simulink model "TargetPosVel"  (R2025a)
settings: Solver=ode4  StartTime=0.0  StopTime=stopTime  FixedStep=timeStep  RelTol=1e-3
values from neighbouring files (symbols this model uses):
  rand_vec = [0, rand(), rand()]    [model_parameters.m]
undefined symbols (not defined in the file or in its folder): angular_rate_noise_ON, angular_rate_noise_power, c, CD, dayValue, dimx, dimz, hourValue, I, I_W, IAU, K_optics, kd, kq, max_h, max_t, minuteValue, mu_E, Omega_E, Phi, pointing_body, q, quat0, quaternion_bias, quaternion_noise_ON, quaternion_sigma, R_E, rcp, res_dipole, secondValue, sma, timeStep, w0, WMM2020, yearValue
libraries: aerolibutil x19, matrix_library x10, aerolibtransform2 x8, vrlib x5, simulink x1, sharedTrackingLibrary x1, aerolibatmos2 x1, aerolibgravity2 x1, sharedtransform x1, sensorgpslib x1, visionsources x1
(part 2 of 2)

== system TargetPosVel/Main/Attiude Controller/Nadir Pointing Controller/Nadir Pointing/Subsystem ==
  r_ECI : Inport
  v_ECI : Inport  Port=2
  Cross Product : matrix_library/Cross Product
  Cross Product1 : matrix_library/Cross Product
  Gain : Gain  Gain=-1
  Matrix Concatenate : Concatenate  NumInputs=3  Mode=Multidimensional array  ConcatenateDimension=2
  Normalize Vector : vrlib/Utilities/Normalize Vector  maxzero=0
  Normalize Vector1 : vrlib/Utilities/Normalize Vector  maxzero=0
  Transpose : Math  Operator=transpose
  DCM_ECI2orb : Outport
  wires:
  Matrix Concatenate/1 -> Transpose/1
  Normalize Vector1/1 -> Cross Product1/1, Matrix Concatenate/2  "y-axis"
  v_ECI/1 -> Cross Product/2
  Gain/1 -> Matrix Concatenate/3, Cross Product1/2  "z-axis"
  Cross Product/1 -> Normalize Vector1/1  "h = r x v"
  Normalize Vector/1 -> Gain/1
  Cross Product1/1 -> Matrix Concatenate/1  "x-axis"
  r_ECI/1 -> Normalize Vector/1, Cross Product/1
  Transpose/1 -> DCM_ECI2orb/1

== system TargetPosVel/Main/Environmental Torques/Environmental Torques/Magnetic Torque/Subsystem ==
  Xi : Inport
  Clock : Clock
  Demux : Demux  Outputs=3
  Direction Cosine Matrix ECEF to NED : aerolibtransform2/Direction Cosine Matrix ECEF to NED
  ECI Position to LLA : aerolibtransform2/ECI Position to LLA  red=IAU-2000/2006  year=yearValue  month=January  day=1  hour=hourValue  min=minuteValue  sec=secondValue  deltaT=Sec  errorflag=Warning  extraparamflag=off  eunits=Metric (MKS)  earthmodel=WGS84  flat=1/298.257223563  eqradius=6378137
      settings: AttributesFormatString=%<red>
  Gain : Gain  Gain=1e-9
  Matrix Multiply : Product  Multiplication=Matrix(*)
  Mux : Mux  Inputs=2
  Selector : Selector  InputPortWidth=3  IndexOptions=Index vector (dialog)  Indices=[3 1 2]  OutputSizes=1
  Transpose : Math  Operator=transpose
  World Magnetic Model : aerolibgravity2/World Magnetic Model  model=WMM2020 (2020-2025)  customFile='WMM2020.COF'  units=Metric (MKS)  time_in=off  month=January  day=1  year=yearValue  action=Error  h_out=off  dec_out=off  inc_out=off  ti_out=off
  MagField_ECEF : Outport
  wires:
  Matrix Multiply/1 -> MagField_ECEF/1
  Demux/3 -> Mux/2, World Magnetic Model/3
  ECI Position to LLA/1 -> Selector/1
  Mux/1 -> Direction Cosine Matrix ECEF to NED/1
  World Magnetic Model/1 -> Gain/1
  Transpose/1 -> Matrix Multiply/1  "DCM_NED2ECEF"
  Selector/1 -> Demux/1
  Gain/1 -> Matrix Multiply/2
  Demux/1 -> World Magnetic Model/1
  Direction Cosine Matrix ECEF to NED/1 -> Transpose/1
  Demux/2 -> Mux/1, World Magnetic Model/2
  Xi/1 -> ECI Position to LLA/1
  Clock/1 -> ?

== matlab function TargetPosVel/Quaternion Noise/MATLAB Function ==
  data: quaternion_sigma input; angle_noise output
function angle_noise = fcn(quaternion_sigma)

% Different simulations use the same seed. OK for reproducibility but not
% good for montecarlo.
noise = randn(2,1)*quaternion_sigma/3600*pi/180*2;
angle_noise = [0; noise];

== matlab function TargetPosVel/Target Position and Velocity - Ideal World/Pixel shift/UV calculation/MATLAB Function ==
  data: img input size=[1200,1920,3]; u input size=1; original_img output size=[1200,1920,3]; v input size=1; shifted_img output size=[1200,1920,3]
function [original_img, shifted_img] = img_shift(img, u, v)

shifted_img  = imtranslate(img, [u,v]);
original_img = img;

end

== matlab function TargetPosVel/Main/Spacecraft Dynamics/GPS/V from ECI to NED/MATLAB Function1 ==
  data: X_icrf input; Reci2ned output
function Reci2ned = ECI2NED(X_icrf)

Reci2ned = eci2ned(X_icrf);

== matlab function TargetPosVel/Target Position and Velocity - Ideal World/Pixel shift/UV calculation/Optical Flow ==
  data: frame1 input size=[1200,1920,3]; u_est output size=1; frame2 input size=[1200,1920,3]; v_est output size=1; precFactor input
function [u_est, v_est] = motion_estimation(frame1, frame2, precFactor)

% Motion estimation between two frames through cross correlation. This code
% gives the same precision as the FFT upsampled cross correlation in a
% small fraction of the computation time and with reduced memory 
% requirements. It obtains an initial estimate of the crosscorrelation peak
% by an FFT and then refines the shift estimation by upsampling the DFT
% only in a small neighborhood of that estimate by means of a 
% matrix-multiply DFT. With this procedure all the image points are used to
% compute the upsampled crosscorrelation.

%% Preprocessing
f = im2single(im2gray(frame1));
g = im2single(im2gray(frame2));

% winRows    = 240;
% winCols    = 384;
% windowSize = [winRows, winCols];
% C          = SelectRegionEdges(f, windowSize);
% 
% f = im2single(f(C(1):C(1)+winRows-1, C(2):C(2)+winCols-1));
% g = im2single(g(C(1):C(1)+winRows-1, C(2):C(2)+winCols-1));

H1 = hann(size((f), 1));
H2 = hann(size((f), 2));

hannWindow = H1*H2';

f = f.*hannWindow;
g = g.*hannWindow;

img1ft = fft2(f);
img2ft = fft2(g);

%% Start with precFactor == 1 to get an integer shift between images
[nr, nc] = size(f);

Nr = ifftshift(-fix(nr/2):ceil(nr/2)-1);
Nc = ifftshift(-fix(nc/2):ceil(nc/2)-1);

% Calculate the cross correlation function between the two images
crossCorr    = ifft2((img2ft.*conj(img1ft))./abs(img2ft.*conj(img1ft)));
abscrossCorr = abs(crossCorr);

[~, maxIndex] = max(abscrossCorr(:)); % linear index of max
[row_shift, col_shift] = ind2sub(size(abscrossCorr), maxIndex);

% Change shifts so that they represent relative shifts and not indices
row_shift = Nr(row_shift);
col_shift = Nc(col_shift);

%% If precision factor is higher than 1, proceed with subpixel refinement
if precFactor >= 2
    %%% DFT computation %%%
    % Center of output array at dftshift+1
    dftshift = fix(ceil(precFactor*1.5)/2);

    % Matrix multiply DFT around the current shift estimate
    crossCorr = conj(dftups((img1ft.*conj(img2ft)), ...
                            ceil(precFactor*1.5), ...
                            ceil(precFactor*1.5), ...
                            precFactor, ...
                            dftshift - row_shift*precFactor, ...
                            dftshift - col_shift*precFactor));

    % Locate maximum and map back to original pixel grid 
    abscrossCorr = abs(crossCorr);

    [~, maxIndex] = max(abscrossCorr(:));       % linear index of max
    [rloc, cloc] = ind2sub(size(abscrossCorr), maxIndex);
    rloc         = rloc - dftshift - 1;
    cloc         = cloc - dftshift - 1;
    
    % Divide rloc and cloc by precFactor to get back to original unit pixel
    % dimensions and sum to the initial integer estimate
    row_shift = row_shift + rloc/precFactor;
    col_shift = col_shift + cloc/precFactor;
end

%% Image final shifts
u_est = col_shift;
v_est = row_shift;

end

%% Fourier Transform Up-sampling
function out = dftups(in, nor, noc, precFactor, roff, coff)

% Upsampled DFT by matrix multiplies, can compute an upsampled DFT in just
% a small region.
% 
% Inputs:
% - precFactor: Precision factor.
% - nor, noc:   Number of pixels in the output upsampled DFT, in units of 
%               upsampled pixels.
% - roff, coff: Row and column offsets, allow to shift the output array to
%               a region of interest on the DFT.
%
% Receives DC in upper left corner, image center must be in (1, 1) 
%
% This code is intended to provide the same result as if the following
% operations were performed:
%
%   1. Embed the array in an array that is 'precFactor' times larger in 
%      each dimension. ifftshift to bring the center of the image to (1,1).
%   2. Take the FFT of the larger array
%   3. Extract an [nor, noc] region of the result. Starting with the 
%      [roff+1 coff+1] element.
%
% It achieves this result by computing the DFT in the output array without
% the need to zeropad. Much faster and memory efficient than the 
% zero-padded  FFT approach if [nor, noc] are much smaller than 
% [nr*usfac, nc*usfac]

[nr, nc] = size(in);

% Compute kernels and obtain DFT by matrix products
kernc = exp((-1i*2*pi/(nc*precFactor))*(ifftshift(0:nc-1).' - floor(nc/2) )*((0:noc-1) - coff));
kernr = exp((-1i*2*pi/(nr*precFactor))*((0:nor-1).' - roff)*(ifftshift(0:nr-1) - floor(nr/2)));

out = kernr*in*kernc;

end

% %% Select region of interest based on number of edges in the image
% function TopLeftAngle = SelectRegionEdges(img, windowSize)
% 
% edgeMap = edge(img, 'Canny');
% 
% windowRows = windowSize(1);
% windowCols = windowSize(2);
% 
% [imgRows, imgCols] = size(img);
% 
% % Region top left angle in the original image (initialization)
% TopLeftAngle = [1, 1];
% 
% % Edge density initialization
% maxDensity = 0;
% 
% for i = 1:windowRows/2:imgRows - windowRows
%     for j = 1:windowCols/2:imgCols - windowCols
%         % Extract the current window
%         Window = edgeMap(i:i+windowRows-1, j:j+windowCols-1);
% 
%         % Find number of edges in the selected region
%         edgeDensity = sum(Window(:));
% 
%         % Update the region center if the new value is higher than the 
%         % previous computed one
%         if edgeDensity > maxDensity
%             maxDensity = edgeDensity;
%             TopLeftAngle = [i, j];
% 
%         end
%     end
% end
% end

== matlab function TargetPosVel/Target Position and Velocity - Ideal World/LOS Calculations/MATLAB Function ==
  data: earthR input; rho output; Rsat_eci input; LOS_hat_eci input
function rho = RHO(earthR,Rsat_eci,LOS_hat_eci)

rho = sphere_intersection(earthR',Rsat_eci',LOS_hat_eci');

== matlab function TargetPosVel/Main/Spacecraft Dynamics/Quaternion kinematics/MATLAB Function ==
  data: omega input; OMEGA output
function OMEGA = buildMatrix(omega)

OMEGA = [   0      -omega(1)  -omega(2)  -omega(3);
         omega(1)      0       omega(3)  -omega(2);
         omega(2)  -omega(3)      0       omega(1);
         omega(3)   omega(2)  -omega(1)      0    ];

end

== matlab function TargetPosVel/Target Position and Velocity - GPS corrupted/LOS Calculations/MATLAB Function ==
  data: earthR input; rho output; Rsat_eci input; LOS_hat_eci input
function rho = RHO(earthR,Rsat_eci,LOS_hat_eci)

rho = sphere_intersection(earthR',Rsat_eci',LOS_hat_eci');

== matlab function TargetPosVel/Target Position and Velocity - GPS corrupted/LOS Calculations/MATLAB Function1 ==
  data: Rsat_eci input; Vtar_eci output; Vsat_eci input; rho input; LOS_hat_eci input; Wsat_eci input; rho_dot output
function [Vtar_eci, rho_dot] = TAR_VELOCITY(Rsat_eci,Vsat_eci,rho,LOS_hat_eci,Wsat_eci)

[Vtar_eci, rho_dot] = target_velocity(rho,LOS_hat_eci',Rsat_eci',Vsat_eci',Wsat_eci');

== matlab function TargetPosVel/Target Position and Velocity - Ideal World/LOS Calculations/MATLAB Function1 ==
  data: Rsat_eci input; Vtar_eci output; Vsat_eci input; rho input; LOS_hat_eci input; Wsat_eci input; rho_dot output
function [Vtar_eci, rho_dot] = TAR_VELOCITY(Rsat_eci,Vsat_eci,rho,LOS_hat_eci,Wsat_eci)

[Vtar_eci, rho_dot] = target_velocity(rho,LOS_hat_eci',Rsat_eci',Vsat_eci',Wsat_eci');

== matlab function TargetPosVel/Estimation Filter/EKF_rho/MATLAB Function1 ==
  data: Rsat_eci input; Vtar_eci output; Vsat_eci input; LOS_hat_eci input; Wsat_eci input; rho input; rho_dot output
function [Vtar_eci, rho_dot] = TAR_VELOCITY(Rsat_eci,Vsat_eci,LOS_hat_eci,Wsat_eci,rho)

[Vtar_eci, rho_dot] = target_velocity(rho,LOS_hat_eci',Rsat_eci',Vsat_eci',Wsat_eci');
